simulink model "Track"  (R2020b)
settings: Solver=VariableStepAuto  StartTime=0.0  StopTime=tm  RelTol=1e-3
values from neighbouring files (symbols this model uses):
  A = [0,1; 1,1]    [Track_m.m]
  B = [0;1]    [Track_m.m]
  C = [1,0]    [Track_m.m]
  w = 1    [Track_m.m]
undefined symbols (not defined in the file or in its folder): Ac, Bc, K, Kc
settings Model: Creator=huang  LastModifiedBy=huang

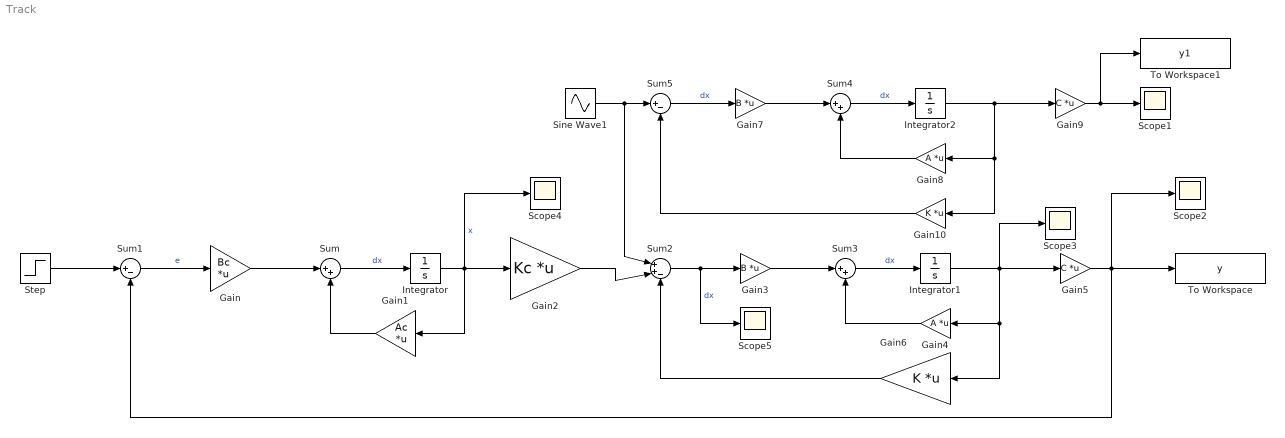
== system Track ==
  Gain : Gain  Gain=Bc  Multiplication=Matrix(K*u)
  Gain1 : Gain  Gain=Ac  Multiplication=Matrix(K*u)
  Gain10 : Gain  Gain=K  Multiplication=Matrix(K*u)
  Gain2 : Gain  Gain=Kc  Multiplication=Matrix(K*u)
  Gain3 : Gain  Gain=B  Multiplication=Matrix(K*u)
  Gain4 : Gain  Gain=A  Multiplication=Matrix(K*u)
  Gain5 : Gain  Gain=C  Multiplication=Matrix(K*u)
  Gain6 : Gain  Gain=K  Multiplication=Matrix(K*u)
  Gain7 : Gain  Gain=B  Multiplication=Matrix(K*u)
  Gain8 : Gain  Gain=A  Multiplication=Matrix(K*u)
  Gain9 : Gain  Gain=C  Multiplication=Matrix(K*u)
  Integrator : Integrator
  Integrator1 : Integrator
  Integrator2 : Integrator
  Scope{1..5} (5 alike) : Scope
  Sine Wave1 : Sin  Amplitude=100  Frequency=w  SampleTime=0
  Step : Step  Time=0  SampleTime=0
  Sum : Sum  Inputs=|++
  Sum1 : Sum  Inputs=|+-
  Sum2 : Sum  Inputs=|++-
  Sum3 : Sum  Inputs=|++
  Sum4 : Sum  Inputs=|++
  Sum5 : Sum  Inputs=|+-
  To Workspace : ToWorkspace  VariableName=y  SampleTime=-1
      settings: Save2DSignal=2-D array (concatenate along first dimension)
  To Workspace1 : ToWorkspace  VariableName=y1  SampleTime=-1
      settings: Save2DSignal=2-D array (concatenate along first dimension)
  wires:
  Gain2/1 -> Sum2/2
  Gain5/1 -> Scope2/1, To Workspace/1, Sum1/2
  Sum2/1 -> Scope5/1, Gain3/1  "dx"
  Gain4/1 -> Sum3/2
  Gain/1 -> Sum/1
  Gain1/1 -> Sum/2
  Sum/1 -> Integrator/1  "dx"
  Sum3/1 -> Integrator1/1  "dx"
  Gain3/1 -> Sum3/1
  Integrator1/1 -> Scope3/1, Gain5/1, Gain6/1, Gain4/1
  Integrator/1 -> Scope4/1, Gain2/1, Gain1/1  "x"
  Gain6/1 -> Sum2/3
  Step/1 -> Sum1/1
  Sum1/1 -> Gain/1  "e"
  Gain10/1 -> Sum5/2
  Sine Wave1/1 -> Sum2/1, Sum5/1
  Gain9/1 -> To Workspace1/1, Scope1/1
  Gain8/1 -> Sum4/2
  Gain7/1 -> Sum4/1
  Integrator2/1 -> Gain8/1, Gain10/1, Gain9/1
  Sum4/1 -> Integrator2/1  "dx"
  Sum5/1 -> Gain7/1  "dx"
